simulink model "pendulum_model"  (R2016b)
settings: Solver=VariableStepAuto  StartTime=0.0  StopTime=100.0  MaxStep=0.01  RelTol=1e-3
values from neighbouring files (symbols this model uses):
  b = 0.1    [pendulum.m]
  g = 9.81    [pendulum.m]
  l = 1    [pendulum.m]
  m = 1    [pendulum.m]
libraries: simulink_extras x1
settings Model: Creator=danii  LastModifiedBy=danii

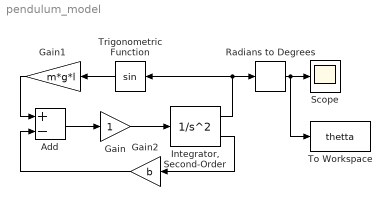
== system pendulum_model ==
  Add : Sum  Inputs=+-
  Gain : Gain
  Gain1 : Gain  Gain=m*g*l
  Gain2 : Gain  Gain=b
  "Integrator, Second-Order" : SecondOrderIntegrator  ICX=0.01
  Radians to Degrees : simulink_extras/Transformations/Radians to Degrees
  Scope : Scope
  To Workspace : ToWorkspace  VariableName=thetta  SampleTime=-1
  Trigonometric Function : Trigonometry
  wires:
  Gain/1 -> "Integrator, Second-Order"/1
  "Integrator, Second-Order"/1 -> Radians to Degrees/1, Trigonometric Function/1
  Trigonometric Function/1 -> Gain1/1
  Gain1/1 -> Add/1
  "Integrator, Second-Order"/2 -> Gain2/1
  Gain2/1 -> Add/2
  Add/1 -> Gain/1
  Radians to Degrees/1 -> To Workspace/1, Scope/1
